simulink model "VanDerPol"  (R2014b)
settings: Solver=ode45  StartTime=0.0  StopTime=10.0  RelTol=1e-3
values from neighbouring files (symbols this model uses):
  mu = 7    [Run_VanDerPol.m]
undefined symbols (not defined in the file or in its folder): param
settings Model: Creator=Arek  LastModifiedBy=Arek

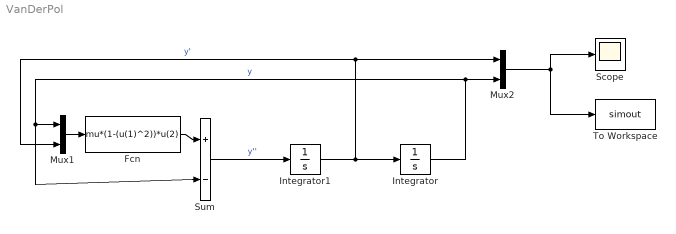
== system VanDerPol ==
  Fcn : Fcn  Expr=mu*(1-(u(1)^2))*u(2)
  Integrator : Integrator  InitialCondition=param.ic(2)
  Integrator1 : Integrator  InitialCondition=param.ic(1)
  Mux1 : Mux  Inputs=2
  Mux2 : Mux  Inputs=2
  Scope : Scope
      settings: ShowLegends=on
  Sum : Sum  Inputs=+|-
  To Workspace : ToWorkspace  VariableName=simout  SaveFormat=Timeseries  SampleTime=-1
  wires:
  Integrator1/1 -> Integrator/1, Mux1/2, Mux2/1  "y'"
  Sum/1 -> Integrator1/1  "y''"
  Fcn/1 -> Sum/1
  Integrator/1 -> Sum/2, Mux1/1, Mux2/2  "y"
  Mux1/1 -> Fcn/1
  Mux2/1 -> Scope/1, To Workspace/1
